simulink model "train_model_sfunction"  (Simulink 8.9)
settings: Solver=FixedStepDiscrete  StartTime=0.0  StopTime=150  FixedStep=1  RelTol=1e-3
libraries: simulink x6, sldvlib x1
settings Model: Creator=Natasha  LastModifiedBy=Natasha
settings DataIOCC: LimitDataPoints=off  SaveFormat=Dataset  SignalLoggingSaveFormat=Dataset  ReturnWorkspaceOutputs=on
settings OptimizationCC: LifeSpan=auto
settings DebuggingCC: UnderspecifiedInitializationDetection=Simplified  MergeDetectMultiDrivingBlocksExec=error  FcnCallInpInsideContextMsg=error  StateNameClashWarn=none  SFUnexpectedBacktrackingDiag=error  SFNoUnconditionalDefaultTransitionDiag=error  SFExecutionAtInitializationDiag=warning
settings HardwareCC: ProdBitPerPointer=64  ProdBitPerSizeT=64  ProdBitPerPtrDiffT=64  ProdLargestAtomicFloat=Float  ProdIntDivRoundTo=Zero  ProdEndianess=LittleEndian  ProdWordSize=64  ProdHWDeviceType=Intel->x86-64 (Windows64)
settings ModelReferenceCC: PropagateSignalLabelsOutOfModel=on
settings SFSimCC: SimUseLocalCustomCode=on
settings RTWCC: RTWUseLocalCustomCode=on
settings GRTTargetCC: TargetLangStandard=C99 (ISO)  GeneratePreprocessorConditionals=Use local settings  CombineOutputUpdateFcns=on  GRTInterface=off
settings ConfigComp: CovMetricSettings=dwe  CovHtmlReporting=off  CovSaveCumulativeToWorkspaceVar=off  CovSaveSingleToWorkspaceVar=off  CovExternalEMLEnable=on

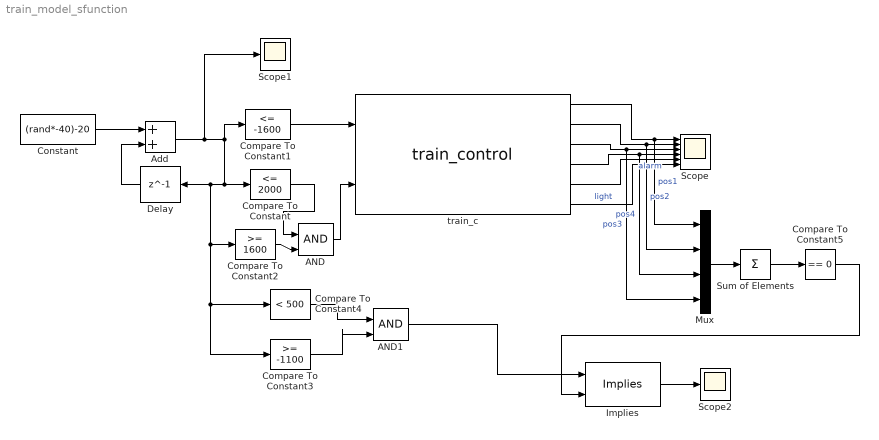
== system train_model_sfunction ==
  AND : Logic  IconShape=distinctive  AllPortsSameDT=off  OutDataTypeStr=boolean
  AND1 : Logic  IconShape=distinctive  AllPortsSameDT=off  OutDataTypeStr=boolean
  Add : Sum
  Compare To Constant : simulink/Logic and Bit Operations/Compare To Constant  relop=<=  const=2000  OutDataTypeStr=boolean
  Compare To Constant1 : simulink/Logic and Bit Operations/Compare To Constant  relop=<=  const=-1600  OutDataTypeStr=boolean
  Compare To Constant2 : simulink/Logic and Bit Operations/Compare To Constant  relop=>=  const=1600  OutDataTypeStr=boolean
  Compare To Constant3 : simulink/Logic and Bit Operations/Compare To Constant  relop=>=  const=-1100  OutDataTypeStr=boolean
  Compare To Constant4 : simulink/Logic and Bit Operations/Compare To Constant  relop=<  const=500  OutDataTypeStr=boolean
  Compare To Constant5 : simulink/Logic and Bit Operations/Compare To Constant  relop===  const=0  OutDataTypeStr=boolean
  Constant : Constant  Value=(rand*-40)-20
  Delay : Delay  DelayLength=1  InitialCondition=2500  UseCircularBuffer=on
  Implies : sldvlib/Verification Utilities/Implies
      settings: SourceProductName=Simulink  SourceProductBaseCode=SL
  Mux : Mux
  Scope : Scope  NumInputPorts=6
  Scope1 : Scope
  Scope2 : Scope
  Sum of Elements : Sum  Inputs=+
  train_c : S-Function  InitFcn=try, set_param(gcb,'FunctionName','train_control'), end  FunctionName=train_control  SFunctionModules=train_control_wrapper  WizardData=DataTag1  SFunctionDeploymentMode=off  EnableBusSupport=off  mask(S-Function Builder){}
      mask help: Simulink:masks:SFunctionBuilder_MD
      mask init:
      | val = [[.9  0.75 0.75 1 1 .9 .9 1]',[1 1 0.75 0.75 .9 .9 1 .9]'];try , sys = get_param(gcb,'SfunBuilderFcnName');if isempty(sys), sys = get_param(gcb,'FunctionName'); end,catch, sys = get_param(gcb,'FunctionName'); end
      settings: CopyFcn=set_param(gcbh,'LinkStatus','none')  PreSaveFcn=try, set_param(gcb,'FunctionName','train_control'), end  OpenFcn=sfunctionwizard(gcbh)
      mask Display: plot(val(:,1),val(:,2)),disp(sys), port_label('input',1,'exited1'), port_label('input',2,'entered1'), port_label('output',1,'pos1'), port_label('output',2,'pos2'), port_label('output',3,'pos3'), port_label('output',4,'pos4'), port_label('output',5,'alarm1'), port_label('output',6,'light')
  wires:
  Delay/1 -> Add/2
  Constant/1 -> Add/1
  Add/1 -> Scope1/1, Compare To Constant1/1, Compare To Constant/1, Compare To Constant3/1, Compare To Constant4/1, Compare To Constant2/1, Delay/1
  Compare To Constant1/1 -> train_c/1
  Compare To Constant2/1 -> AND/2
  Compare To Constant/1 -> AND/1
  AND/1 -> train_c/2
  train_c/1 -> Mux/1, Scope/1  "pos1"
  train_c/2 -> Mux/2, Scope/2  "pos2"
  train_c/3 -> Mux/4, Scope/3  "pos3"
  train_c/4 -> Mux/3, Scope/4  "pos4"
  train_c/5 -> Scope/5  "alarm"
  train_c/6 -> Scope/6  "light"
  Compare To Constant3/1 -> AND1/2
  Compare To Constant4/1 -> AND1/1
  Mux/1 -> Sum of Elements/1
  Sum of Elements/1 -> Compare To Constant5/1
  AND1/1 -> Implies/1
  Compare To Constant5/1 -> Implies/2
  Implies/1 -> Scope2/1
